simulink model "AC_Voltage_Control_3phase_IM"  (R2025a)
settings: Solver=ode23t  StartTime=0.0  StopTime=5  FixedStep=0.00001  MaxStep=10e-6  RelTol=1e-3  EnableMultiTasking=on
undefined symbols (not defined in the file): DiscIntNeverNeededParam
libraries: spsDetailedThyristorLib x6, spsVoltageMeasurementLib x6, spsACVoltageSourceLib x3, spsAsynchronousMachineSIUnitsLib x1, powerlib_extras x1, spsSeriesRLCBranchLib x1, spsThreePhaseVIMeasurementLib x1, sps_lib x1
settings Model: Creator=jagan  LastModifiedBy=Shubham Raj Gupta
settings SolverCC: ZeroCrossControl=DisableAll  ZeroCrossAlgorithm=Non-adaptive  AlgebraicLoopSolver=TrustRegion
settings DataIOCC: LimitDataPoints=on  SaveFormat=Array  SignalLoggingSaveFormat=ModelDataLogs  ReturnWorkspaceOutputs=off
settings OptimizationCC: ExpressionDepthLimit=2147483647.0  InitFltsAndDblsToZero=on  LifeSpan=inf
settings DebuggingCC: SaveWithParameterizedLinksMsg=none  UnderspecifiedInitializationDetection=Classic  MergeDetectMultiDrivingBlocksExec=none  SignalResolutionControl=TryResolveAllWithWarning  SolverPrmCheckMsg=warning  MultiTaskDSMMsg=warning  MultiTaskCondExecSysMsg=none  FcnCallInpInsideContextMsg=warning  UnconnectedInputMsg=warning  UnconnectedOutputMsg=warning  UnconnectedLineMsg=warning  StateNameClashWarn=warning  SFUnexpectedBacktrackingDiag=warning  SFNoUnconditionalDefaultTransitionDiag=warning  SFExecutionAtInitializationDiag=none  ArithmeticOperatorsInVariantConditions=warning
settings HardwareCC: ProdBitPerPointer=32.0  ProdBitPerSizeT=32.0  ProdBitPerPtrDiffT=32.0  ProdLargestAtomicFloat=None  ProdIntDivRoundTo=Undefined  ProdEndianess=Unspecified  ProdWordSize=32.0  ProdHWDeviceType=32-bit Generic
settings ModelReferenceCC: PropagateSignalLabelsOutOfModel=off
settings SFSimCC: SimParseCustomCode=off
settings RTWCC: GPUComputeCapability=3.5
settings CodeAppCC: StateflowObjectComments=on
settings GRTTargetCC: TargetFcnLib=ansi_tfl_tmw.mat  TargetLangStandard=C89/C90 (ANSI)  CombineOutputUpdateFcns=off  GRTInterface=on
settings ConfigComp: CovMetricSettings=dw  CovSaveCumulativeToWorkspaceVar=on  CovSaveSingleToWorkspaceVar=on

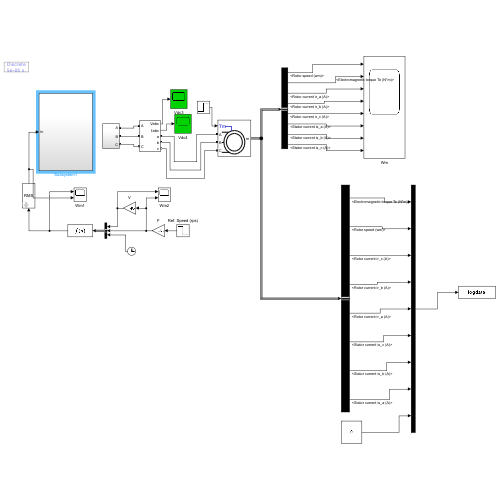
[thumbnail: Simulink's stored preview of the top-level diagram]
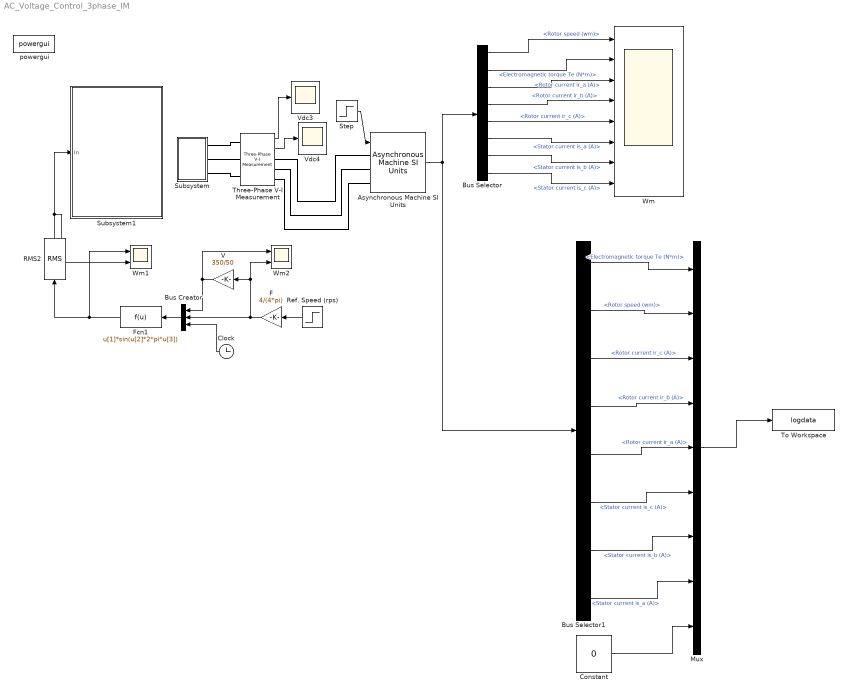
== system AC_Voltage_Control_3phase_IM ==
  Asynchronous Machine SI Units : spsAsynchronousMachineSIUnitsLib/Asynchronous Machine SI Units  RotorType=Squirrel-cage  PresetModel=No  MechanicalLoad=Torque Tm  ShowDetailedParameters=on  ReferenceFrame=Rotor  Units=SI  MeasurementBus=off  NominalParameters=[3730 400 50]  VoltageRatio=1  Stator=[1.115 0.005974]  Rotor=[100 0.005974]  Cage1=[0.4155 0.002066]  Cage2=[0.4168 0.0003495]  Lm=0.2037  Mechanical=[0.02 0.005752 2]  PolePairs=2  InitialConditions="[ 1,0   0,0,0   0,0,0 ]"  SimulateSaturation=off  Saturation=[9.9249,19.6672,38.0377,51.3988,69.2824,105.1337,152.5532,214.2421,303.1917;230, 322, 414, 460, 506, 552, 598, 644, 690]  LoadFlowParameters=0  TsPowergui=0  TsBlock=-1  IterativeModel=Trapezoidal non iterative  IterativeDiscreteModel=Trapezoidal non iterative  Pmec=1.492e+006
  Bus Creator : BusCreator  Inputs=3
  Bus Selector : BusSelector  OutputSignals=Mechanical.Rotor speed (wm),Mechanical.Electromagnetic torque Te (N*m),Rotor measurements.Rotor current ir_a (A),Rotor measurements.Rotor current ir_b (A),Rotor measurements.Rotor current ir_c (A),Stator measurements.Stator current is_a (A),Stator measurements.Stator current is_b (A),Stator measurements.Stator current is_c (A)
  Bus Selector1 : BusSelector  OutputSignals=Mechanical.Electromagnetic torque Te (N*m),Mechanical.Rotor speed (wm),Rotor measurements.Rotor current ir_c (A),Rotor measurements.Rotor current ir_b (A),Rotor measurements.Rotor current ir_a (A),Stator measurements.Stator current is_c (A),Stator measurements.Stator current is_b (A),Stator measurements.Stator current is_a (A)
  Clock : Clock
  Constant : Constant  Value=0
  F : Gain  Gain=4/(4*pi)
  Fcn1 : Fcn  Expr=u[1]*sin(u[2]*2*pi*u[3])
  Mux : Mux  Inputs=9
  RMS2 : powerlib_extras/Measurements/RMS  f1=50
  Ref. Speed (rps) : Step  Time=3  Before=150  After=120  SampleTime=0
  Step : Step  After=3  SampleTime=0
  Subsystem : Subsystem
  Subsystem1 : Subsystem
  Three-Phase V-I Measurement : spsThreePhaseVIMeasurementLib/Three-Phase V-I Measurement  VoltageMeasurement=phase-to-phase  SetLabelV=off  LabelV=Vabc  Vpu=off  VpuLL=off  CurrentMeasurement=yes  SetLabelI=off  LabelI=Iabc  Ipu=off  Pbase=100e6  Vbase=500e3  OutputType=Complex  PhasorSimulation=off  PSBequivalent=0
  To Workspace : ToWorkspace  VariableName=logdata  SampleTime=5e-5
  V : Gain  Gain=350/50
  Vdc3 : Scope
      settings: SampleTime=100e-6  TimeSpan=0.04  ActiveDisplayYMinimum=-700  ActiveDisplayYMaximum=700  DataLoggingVariableName=Ia_3
  Vdc4 : Scope
      settings: SampleTime=100e-6  TimeSpan=1  ActiveDisplayYMinimum=549.65  ActiveDisplayYMaximum=549.82  DataLoggingVariableName=Ia_4
  Wm : Scope  NumInputPorts=8
      settings: ActiveDisplayYMinimum=-300  ActiveDisplayYMaximum=207.4144440126116  DataLoggingVariableName=ScopeData9
  Wm1 : Scope  NumInputPorts=2
      settings: TimeSpan=0.04  ActiveDisplayYMinimum=-350  ActiveDisplayYMaximum=350
  Wm2 : Scope  NumInputPorts=2
      settings: ActiveDisplayYMinimum=332.332  ActiveDisplayYMaximum=367.314  DataLoggingVariableName=ScopeData7
  powergui : sps_lib/powergui  SimulationMode=Discrete  SampleTime=50e-6  frequency=60  Iterations=50  frequencyindice=50  Pbase=100e6  ErrMax=1e-4  UnitsV=kV  UnitsW=MW  buscounter=0  FunctionMessages=off  echomessages=off  EnableUseOfTLC=off  CurrentSourceSwitches=off  DisableSnubberDevices=off  DisableRonSwitches=off  DisableVfSwitches=off  DisplayEquations=off  AutomaticDiscreteSolvers=off  SolverType=Tustin/Backward Euler (TBE)  Interpol=off  ExternalGateDelay=off  methode=off  Ts=0  x0status=blocks  SPID=off  SwTol=0  HookPort=off  NonlinearTolerance=1e-4  nMaxIteration=100  ContinueOnMaxIteration=off  RestoreLinks=warning  ResistiveCurrentMeasurement=off  Frange=[0:2:500]  Ylog=off  Xlog=on  ShowGrid=off  save=off  variable=ZData  structure=0  ZoomFFT=on  StartTime=0.0  cycles=1  DisplayStyle=1  fundamental=60  FreqAxis=off  MaxFrequency=1000  frequencyindicesteady=1  RmsSteady=1  display=off
  wires:
  Bus Creator/1 -> Fcn1/1
  Clock/1 -> Bus Creator/3
  F/1 -> Bus Creator/2, V/1, Wm2/2
  V/1 -> Bus Creator/1, Wm2/1
  Ref. Speed (rps)/1 -> F/1
  Fcn1/1 -> RMS2/1, Wm1/1
  RMS2/1 -> Subsystem1/1(In), Wm1/2
  Step/1 -> Asynchronous Machine SI Units/1
  Asynchronous Machine SI Units/1 -> Bus Selector1/1, Bus Selector/1
  Bus Selector/1 -> Wm/1  "<Rotor speed (wm)>"
  Bus Selector/2 -> Wm/2  "<Electromagnetic torque Te (N*m)>"
  Three-Phase V-I Measurement/1 -> Vdc3/1
  Three-Phase V-I Measurement/2 -> Vdc4/1
  Constant/1 -> Mux/9
  Mux/1 -> To Workspace/1
  Bus Selector1/1 -> Mux/1  "<Electromagnetic torque Te (N*m)>"
  Bus Selector1/2 -> Mux/2  "<Rotor speed (wm)>"
  Bus Selector1/3 -> Mux/3  "<Rotor current ir_c (A)>"
  Bus Selector1/4 -> Mux/4  "<Rotor current ir_b (A)>"
  Bus Selector1/5 -> Mux/5  "<Rotor current ir_a (A)>"
  Bus Selector1/6 -> Mux/6  "<Stator current is_c (A)>"
  Bus Selector1/7 -> Mux/7  "<Stator current is_b (A)>"
  Bus Selector1/8 -> Mux/8  "<Stator current is_a (A)>"
  Bus Selector/3 -> Wm/3  "<Rotor current ir_a (A)>"
  Bus Selector/4 -> Wm/4  "<Rotor current ir_b (A)>"
  Bus Selector/5 -> Wm/5  "<Rotor current ir_c (A)>"
  Bus Selector/6 -> Wm/6  "<Stator current is_a (A)>"
  Bus Selector/7 -> Wm/7  "<Stator current is_b (A)>"
  Bus Selector/8 -> Wm/8  "<Stator current is_c (A)>"
  connections:
  Three-Phase V-I Measurement/LConn1 -- Subsystem/RConn1
  Subsystem/RConn2 -- Three-Phase V-I Measurement/LConn2
  Three-Phase V-I Measurement/LConn3 -- Subsystem/RConn3
  Three-Phase V-I Measurement/RConn1 -- Asynchronous Machine SI Units/LConn1
  Asynchronous Machine SI Units/LConn2 -- Three-Phase V-I Measurement/RConn2
  Three-Phase V-I Measurement/RConn3 -- Asynchronous Machine SI Units/LConn3

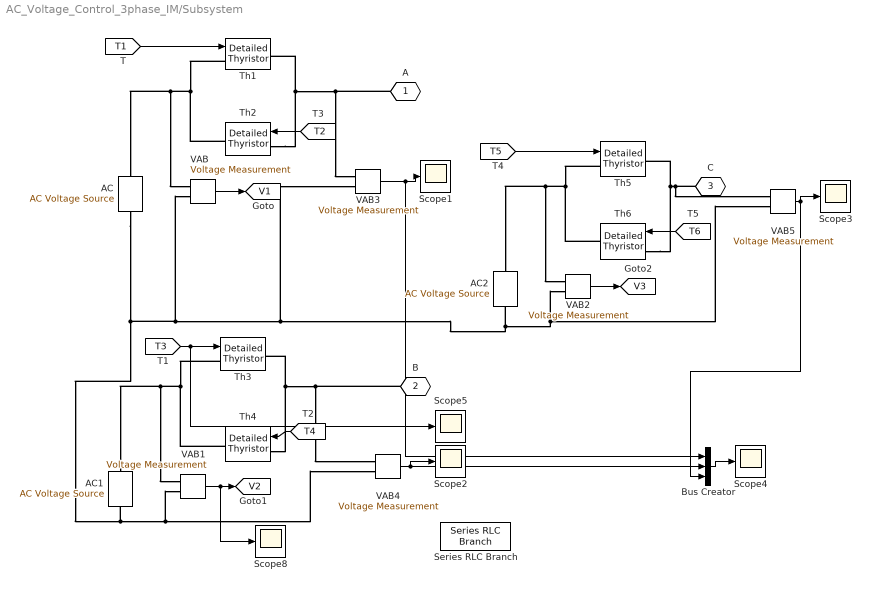
== system AC_Voltage_Control_3phase_IM/Subsystem ==
  AC : spsACVoltageSourceLib/AC Voltage Source  Amplitude=250*1.414  Phase=0  Frequency=50  SampleTime=0  Measurements=None  BusType=swing  Pref=10e3  Qref=0  Qmin=-inf  Qmax=+inf
  AC1 : spsACVoltageSourceLib/AC Voltage Source  Amplitude=250*1.414  Phase=240  Frequency=50  SampleTime=0  Measurements=None  BusType=swing  Pref=10e3  Qref=0  Qmin=-inf  Qmax=+inf
  AC2 : spsACVoltageSourceLib/AC Voltage Source  Amplitude=250*1.414  Phase=120  Frequency=50  SampleTime=0  Measurements=None  BusType=swing  Pref=10e3  Qref=0  Qmin=-inf  Qmax=+inf
  Bus Creator : BusCreator  Inputs=3
  Scope{1..5,8} (6 alike) : Scope
      Scope1 settings: TimeSpan=0.04  ActiveDisplayYMinimum=-300  ActiveDisplayYMaximum=300  DataLoggingVariableName=ScopeData2
      Scope2 settings: TimeSpan=0.04  ActiveDisplayYMinimum=-400  ActiveDisplayYMaximum=400  DataLoggingVariableName=ScopeData3
      Scope3 settings: TimeSpan=0.04  ActiveDisplayYMinimum=-400  ActiveDisplayYMaximum=400  DataLoggingVariableName=ScopeData4
      Scope4 settings: TimeSpan=0.04  ActiveDisplayYMinimum=-400  ActiveDisplayYMaximum=400  DataLoggingVariableName=ScopeData5
      Scope5 settings: TimeSpan=0.04  ActiveDisplayYMinimum=0  ActiveDisplayYMaximum=1  DataLoggingVariableName=ScopeData6
      Scope8 settings: TimeSpan=0.04  ActiveDisplayYMinimum=-400  ActiveDisplayYMaximum=400  DataLoggingVariableName=ScopeData10
  Series RLC Branch : spsSeriesRLCBranchLib/Series RLC Branch  LConnTagsString=__new0  RConnTagsString=__new0  BranchType=RLC  Resistance=1  Inductance=1e-3  SetiL0=off  InitialCurrent=0  Capacitance=1e-6  Setx0=off  InitialVoltage=0  Measurements=None
  Th{1..6} (6 alike) : spsDetailedThyristorLib/Detailed Thyristor  Ron=0.001  Lon=0  Vf=0.8  IL=0.1  Tq=100e-6  IC=0  Rs=500  Cs=250e-9  Measurements=off
      settings: LibrarySourceBlock=sps_lib/Power Electronics/Detailed Thyristor
  VAB{,1..5} (6 alike) : spsVoltageMeasurementLib/Voltage Measurement  PhasorSimulation=off  OutputType=Complex  PSBequivalent=0
  A : PMIOPort  Tag=PMCPort  Side=Right
  B : PMIOPort  Tag=PMCPort  Port=2  Side=Right
  C : PMIOPort  Tag=PMCPort  Port=3  Side=Right
  tag scope: V1=global, V2=global, V3=global
  wires:
  VAB/1 -> [V1]
  [T1] -> Th1/1
  [T2] -> Th2/1
  VAB1/1 -> [V2], Scope8/1
  [T3] -> Scope5/1, Th3/1
  [T4] -> Th4/1
  VAB2/1 -> [V3]
  [T5] -> Th5/1
  [T6] -> Th6/1
  VAB3/1 -> Scope1/1, Bus Creator/1
  VAB4/1 -> Scope2/1, Bus Creator/2
  VAB5/1 -> Scope3/1, Bus Creator/3
  Bus Creator/1 -> Scope4/1
  connections:
  Th1/LConn1 -- AC/RConn1 -- VAB/LConn1 -- Th2/RConn1
  Th4/RConn1 -- VAB1/LConn1 -- AC1/RConn1 -- Th3/LConn1
  Th1/RConn1 -- A/RConn1 -- VAB3/LConn1 -- Th2/LConn1
  Th4/LConn1 -- VAB4/LConn1 -- B/RConn1 -- Th3/RConn1
  Th5/LConn1 -- AC2/RConn1 -- VAB2/LConn1 -- Th6/RConn1
  Th5/RConn1 -- C/RConn1 -- VAB5/LConn1 -- Th6/LConn1
  VAB1/LConn2 -- VAB4/LConn2 -- AC1/LConn1 -- AC/LConn1 -- VAB/LConn2 -- VAB3/LConn2 -- AC2/LConn1 -- VAB2/LConn2 -- VAB5/LConn2

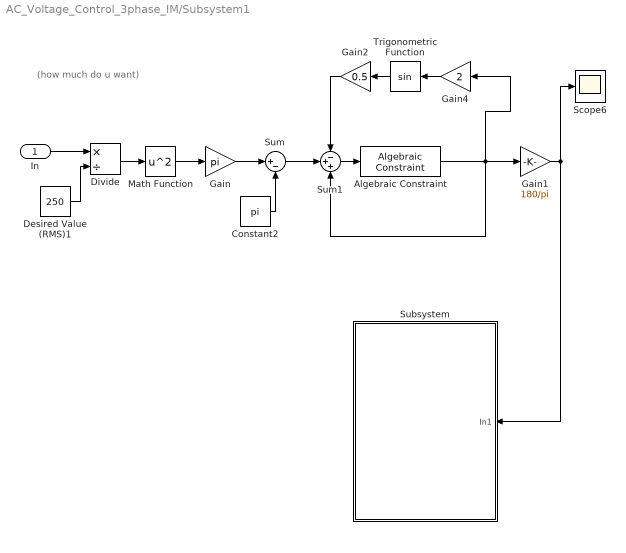
== system AC_Voltage_Control_3phase_IM/Subsystem1 ==
  note: (how much do u want)
  In : Inport
  Algebraic Constraint : AlgebraicConstraint  InitialGuess=pi
  Constant2 : Constant  Value=pi
  Desired Value (RMS)1 : Constant  Value=250
  Divide : Product  Inputs=*/
  Gain : Gain  Gain=pi
  Gain1 : Gain  Gain=180/pi
  Gain2 : Gain  Gain=0.5
  Gain4 : Gain  Gain=2
  Math Function : Math  Operator=square  SignedPower=on
  Scope6 : Scope
      settings: TimeSpan=0.04  ActiveDisplayYMinimum=26.65  ActiveDisplayYMaximum=27.15
  Subsystem : Subsystem
  Sum : Sum  Inputs=|+-
  Sum1 : Sum  Inputs=-++
  Trigonometric Function : Trigonometry  SampleTime=0.0001
  wires:
  In/1 -> Divide/1
  Divide/1 -> Math Function/1
  Math Function/1 -> Gain/1
  Gain/1 -> Sum/1
  Constant2/1 -> Sum/2
  Sum1/1 -> Algebraic Constraint/1
  Algebraic Constraint/1 -> Sum1/3, Gain1/1, Gain4/1
  Gain4/1 -> Trigonometric Function/1
  Trigonometric Function/1 -> Gain2/1
  Gain2/1 -> Sum1/1
  Sum/1 -> Sum1/2
  Gain1/1 -> Scope6/1, Subsystem/1(In1)
  Desired Value (RMS)1/1 -> Divide/2

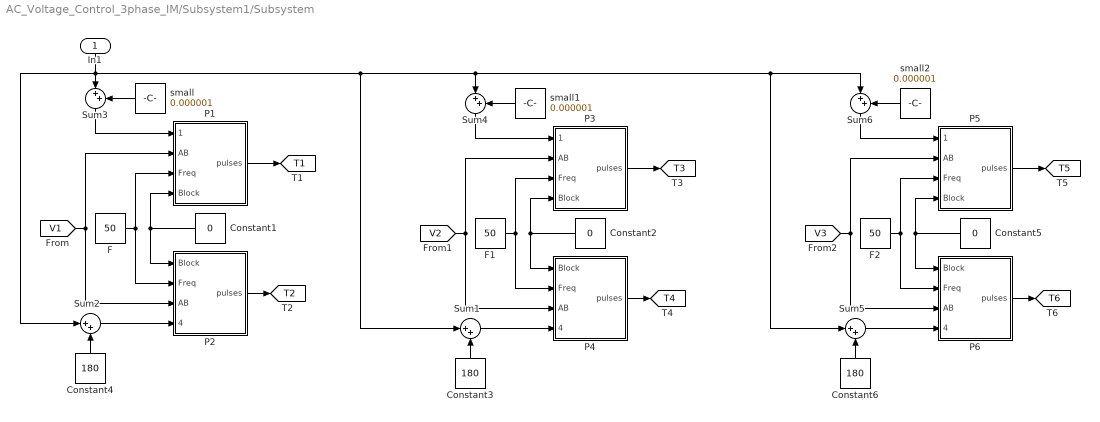
== system AC_Voltage_Control_3phase_IM/Subsystem1/Subsystem ==
  In1 : Inport
  Constant1 : Constant  Value=0
  Constant2 : Constant  Value=0
  Constant3 : Constant  Value=180
  Constant4 : Constant  Value=180
  Constant5 : Constant  Value=0
  Constant6 : Constant  Value=180
  F : Constant  Value=50
  F1 : Constant  Value=50
  F2 : Constant  Value=50
  P1 : Subsystem  AncestorBlock=|  DialogController=POWERSYS.PowerSysDialog  mask(Discrete Synchronized 6-pulse generator){pwidth=10, Double_Pulse=on, Ts=0.0001}
      | powerlib_extras/Discrete 
      | Control Blocks/Discrete Synchronized
      | 6-Pulse Generator
      mask prompts: pwidth "Pulse width (degrees) :"; Double_Pulse "Double pulsing"; Ts "Time step (s) :"
      mask help:
      | Use this block to fire the 6 thyristors of a 6-pulse converter.
      |
      | The output is a vector of 6 pulses (0-1) individually synchronized on the 6 commutation voltages. Pulses are generated alpha degrees after the increasing zero-crossings of the commutation voltages.
      |
      | Input 1 is  the alpha firing signal (degrees).
      | Inputs 2, 3 and 4 are the synchronization voltages AB BC CA which should be in phase with the 3 phase-phase voltages at the converter terminals.
      | Input 5: Frequency of the synchronization voltages (use a constant or the Freq PLL output)
      | Input 6 allows  blocking of the pulses when the applied signal is non zero.
      |
      | When the 'Douple pulsing' option is checked, two pulses are sent to each thyristor: a 1st pulse when the aplha angle is reached, then a 2nd pulse 60 degrees later, when the next thyristor is fired.
      mask init:
      | power_initmask();
      mask Help: This block is part of a subset of blocks in the Extras library that does not have documentation associated with it, other than the block mask description.
      mask Display: plot(0,0,100,100,[80 62 62 47 47 30],[40 40 60 60 40 40]-5)
  P2 : Subsystem  AncestorBlock=|  DialogController=POWERSYS.PowerSysDialog  mask(Discrete Synchronized 6-pulse generator){pwidth=10, Double_Pulse=on, Ts=0.0001}
      | powerlib_extras/Discrete 
      | Control Blocks/Discrete Synchronized
      | 6-Pulse Generator
      mask prompts: pwidth "Pulse width (degrees) :"; Double_Pulse "Double pulsing"; Ts "Time step (s) :"
      mask help:
      | Use this block to fire the 6 thyristors of a 6-pulse converter.
      |
      | The output is a vector of 6 pulses (0-1) individually synchronized on the 6 commutation voltages. Pulses are generated alpha degrees after the increasing zero-crossings of the commutation voltages.
      |
      | Input 1 is  the alpha firing signal (degrees).
      | Inputs 2, 3 and 4 are the synchronization voltages AB BC CA which should be in phase with the 3 phase-phase voltages at the converter terminals.
      | Input 5: Frequency of the synchronization voltages (use a constant or the Freq PLL output)
      | Input 6 allows  blocking of the pulses when the applied signal is non zero.
      |
      | When the 'Douple pulsing' option is checked, two pulses are sent to each thyristor: a 1st pulse when the aplha angle is reached, then a 2nd pulse 60 degrees later, when the next thyristor is fired.
      mask init:
      | power_initmask();
      mask Help: This block is part of a subset of blocks in the Extras library that does not have documentation associated with it, other than the block mask description.
      mask Display: plot(0,0,100,100,[80 62 62 47 47 30],[40 40 60 60 40 40]-5)
  P3 : Subsystem  AncestorBlock=|  DialogController=POWERSYS.PowerSysDialog  mask(Discrete Synchronized 6-pulse generator){pwidth=180, Double_Pulse=on, Ts=0.0001}
      | powerlib_extras/Discrete 
      | Control Blocks/Discrete Synchronized
      | 6-Pulse Generator
      mask prompts: pwidth "Pulse width (degrees) :"; Double_Pulse "Double pulsing"; Ts "Time step (s) :"
      mask help:
      | Use this block to fire the 6 thyristors of a 6-pulse converter.
      |
      | The output is a vector of 6 pulses (0-1) individually synchronized on the 6 commutation voltages. Pulses are generated alpha degrees after the increasing zero-crossings of the commutation voltages.
      |
      | Input 1 is  the alpha firing signal (degrees).
      | Inputs 2, 3 and 4 are the synchronization voltages AB BC CA which should be in phase with the 3 phase-phase voltages at the converter terminals.
      | Input 5: Frequency of the synchronization voltages (use a constant or the Freq PLL output)
      | Input 6 allows  blocking of the pulses when the applied signal is non zero.
      |
      | When the 'Douple pulsing' option is checked, two pulses are sent to each thyristor: a 1st pulse when the aplha angle is reached, then a 2nd pulse 60 degrees later, when the next thyristor is fired.
      mask init:
      | power_initmask();
      mask Help: This block is part of a subset of blocks in the Extras library that does not have documentation associated with it, other than the block mask description.
      mask Display: plot(0,0,100,100,[80 62 62 47 47 30],[40 40 60 60 40 40]-5)
  P4 : Subsystem  AncestorBlock=|  DialogController=POWERSYS.PowerSysDialog  mask(Discrete Synchronized 6-pulse generator){pwidth=180, Double_Pulse=on, Ts=0.0001}
      | powerlib_extras/Discrete 
      | Control Blocks/Discrete Synchronized
      | 6-Pulse Generator
      mask prompts: pwidth "Pulse width (degrees) :"; Double_Pulse "Double pulsing"; Ts "Time step (s) :"
      mask help:
      | Use this block to fire the 6 thyristors of a 6-pulse converter.
      |
      | The output is a vector of 6 pulses (0-1) individually synchronized on the 6 commutation voltages. Pulses are generated alpha degrees after the increasing zero-crossings of the commutation voltages.
      |
      | Input 1 is  the alpha firing signal (degrees).
      | Inputs 2, 3 and 4 are the synchronization voltages AB BC CA which should be in phase with the 3 phase-phase voltages at the converter terminals.
      | Input 5: Frequency of the synchronization voltages (use a constant or the Freq PLL output)
      | Input 6 allows  blocking of the pulses when the applied signal is non zero.
      |
      | When the 'Douple pulsing' option is checked, two pulses are sent to each thyristor: a 1st pulse when the aplha angle is reached, then a 2nd pulse 60 degrees later, when the next thyristor is fired.
      mask init:
      | power_initmask();
      mask Help: This block is part of a subset of blocks in the Extras library that does not have documentation associated with it, other than the block mask description.
      mask Display: plot(0,0,100,100,[80 62 62 47 47 30],[40 40 60 60 40 40]-5)
  P5 : Subsystem  AncestorBlock=|  DialogController=POWERSYS.PowerSysDialog  mask(Discrete Synchronized 6-pulse generator){pwidth=180, Double_Pulse=on, Ts=0.0001}
      | powerlib_extras/Discrete 
      | Control Blocks/Discrete Synchronized
      | 6-Pulse Generator
      mask prompts: pwidth "Pulse width (degrees) :"; Double_Pulse "Double pulsing"; Ts "Time step (s) :"
      mask help:
      | Use this block to fire the 6 thyristors of a 6-pulse converter.
      |
      | The output is a vector of 6 pulses (0-1) individually synchronized on the 6 commutation voltages. Pulses are generated alpha degrees after the increasing zero-crossings of the commutation voltages.
      |
      | Input 1 is  the alpha firing signal (degrees).
      | Inputs 2, 3 and 4 are the synchronization voltages AB BC CA which should be in phase with the 3 phase-phase voltages at the converter terminals.
      | Input 5: Frequency of the synchronization voltages (use a constant or the Freq PLL output)
      | Input 6 allows  blocking of the pulses when the applied signal is non zero.
      |
      | When the 'Douple pulsing' option is checked, two pulses are sent to each thyristor: a 1st pulse when the aplha angle is reached, then a 2nd pulse 60 degrees later, when the next thyristor is fired.
      mask init:
      | power_initmask();
      mask Help: This block is part of a subset of blocks in the Extras library that does not have documentation associated with it, other than the block mask description.
      mask Display: plot(0,0,100,100,[80 62 62 47 47 30],[40 40 60 60 40 40]-5)
  P6 : Subsystem  AncestorBlock=|  DialogController=POWERSYS.PowerSysDialog  mask(Discrete Synchronized 6-pulse generator){pwidth=180, Double_Pulse=on, Ts=0.0001}
      | powerlib_extras/Discrete 
      | Control Blocks/Discrete Synchronized
      | 6-Pulse Generator
      mask prompts: pwidth "Pulse width (degrees) :"; Double_Pulse "Double pulsing"; Ts "Time step (s) :"
      mask help:
      | Use this block to fire the 6 thyristors of a 6-pulse converter.
      |
      | The output is a vector of 6 pulses (0-1) individually synchronized on the 6 commutation voltages. Pulses are generated alpha degrees after the increasing zero-crossings of the commutation voltages.
      |
      | Input 1 is  the alpha firing signal (degrees).
      | Inputs 2, 3 and 4 are the synchronization voltages AB BC CA which should be in phase with the 3 phase-phase voltages at the converter terminals.
      | Input 5: Frequency of the synchronization voltages (use a constant or the Freq PLL output)
      | Input 6 allows  blocking of the pulses when the applied signal is non zero.
      |
      | When the 'Douple pulsing' option is checked, two pulses are sent to each thyristor: a 1st pulse when the aplha angle is reached, then a 2nd pulse 60 degrees later, when the next thyristor is fired.
      mask init:
      | power_initmask();
      mask Help: This block is part of a subset of blocks in the Extras library that does not have documentation associated with it, other than the block mask description.
      mask Display: plot(0,0,100,100,[80 62 62 47 47 30],[40 40 60 60 40 40]-5)
  Sum{1..6} (6 alike) : Sum  Inputs=|++
  small : Constant  Value=0.000001
  small1 : Constant  Value=0.000001
  small2 : Constant  Value=0.000001
  tag scope: T1=global, T2=global, T3=global, T4=global, T5=global, T6=global
  wires:
  Constant4/1 -> Sum2/2
  small/1 -> Sum3/2
  Sum3/1 -> P1/1(alpha_deg)
  Constant1/1 -> P1/4(Block), P2/1(Block)
  F/1 -> P1/3(Freq), P2/2(Freq)
  Sum2/1 -> P2/4(alpha_deg)
  [V1] -> P1/2(AB), P2/3(AB)
  P1/1(pulses) -> [T1]
  P2/1(pulses) -> [T2]
  In1/1 -> Sum3/1, Sum1/1, Sum4/1, Sum6/1, Sum5/1, Sum2/1
  Constant3/1 -> Sum1/2
  small1/1 -> Sum4/2
  Sum4/1 -> P3/1(alpha_deg)
  Constant2/1 -> P4/1(Block), P3/4(Block)
  F1/1 -> P4/2(Freq), P3/3(Freq)
  Sum1/1 -> P4/4(alpha_deg)
  [V2] -> P4/3(AB), P3/2(AB)
  P3/1(pulses) -> [T3]
  P4/1(pulses) -> [T4]
  Constant6/1 -> Sum5/2
  small2/1 -> Sum6/2
  Sum6/1 -> P5/1(alpha_deg)
  Constant5/1 -> P5/4(Block), P6/1(Block)
  F2/1 -> P5/3(Freq), P6/2(Freq)
  Sum5/1 -> P6/4(alpha_deg)
  [V3] -> P5/2(AB), P6/3(AB)
  P5/1(pulses) -> [T5]
  P6/1(pulses) -> [T6]

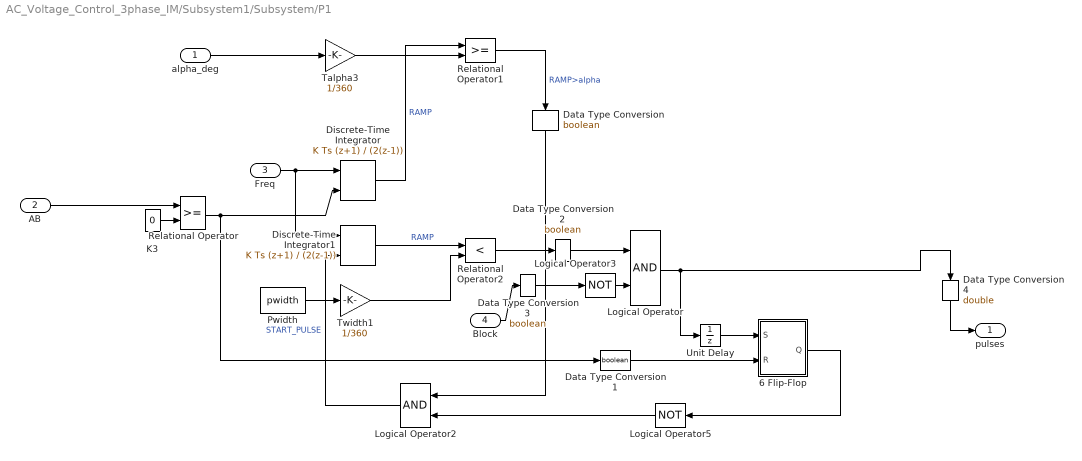
== system AC_Voltage_Control_3phase_IM/Subsystem1/Subsystem/P1 ==
  alpha_deg : Inport
  AB : Inport  Port=2
  Freq : Inport  Port=3
  Block : Inport  Port=4
  6 Flip-Flop : Subsystem
  Data Type Conversion{,1..3} (4 alike) : DataTypeConversion  OutDataTypeStr=boolean
  Data Type Conversion4 : DataTypeConversion  OutDataTypeStr=double
  Discrete-Time Integrator : DiscreteIntegrator  IntegratorMethod=Integration: Trapezoidal  ExternalReset=rising  SampleTime=Ts  ICPrevOutput=DiscIntNeverNeededParam  ICPrevScaledInput=DiscIntNeverNeededParam
  Discrete-Time Integrator1 : DiscreteIntegrator  IntegratorMethod=Integration: Trapezoidal  ExternalReset=rising  SampleTime=Ts  ICPrevOutput=DiscIntNeverNeededParam  ICPrevScaledInput=DiscIntNeverNeededParam
  K3 : Constant  Value=0
  Logical Operator : Logic
  Logical Operator2 : Logic
  Logical Operator3 : Logic  Operator=NOT  Inputs=1
  Logical Operator5 : Logic  Operator=NOT  Inputs=1
  Pwidth : Constant  Value=pwidth
  Relational Operator : RelationalOperator
  Relational Operator1 : RelationalOperator
  Relational Operator2 : RelationalOperator  Operator=<
  Talpha3 : Gain  Gain=1/360  SaturateOnIntegerOverflow=on  OutDataTypeStr=Inherit: Same as input  ParamDataTypeStr=Inherit: Same as input
  Twidth1 : Gain  Gain=1/360  SaturateOnIntegerOverflow=on  OutDataTypeStr=Inherit: Same as input  ParamDataTypeStr=Inherit: Same as input
  Unit Delay : UnitDelay  SampleTime=Ts
  pulses : Outport  InitialOutput=0
  wires:
  Data Type Conversion4/1 -> pulses/1
  Data Type Conversion3/1 -> Logical Operator3/1
  Block/1 -> Data Type Conversion3/1
  Data Type Conversion2/1 -> Logical Operator/1
  Relational Operator2/1 -> Data Type Conversion2/1
  Data Type Conversion1/1 -> 6 Flip-Flop/2(R)
  Data Type Conversion/1 -> Logical Operator2/1
  Relational Operator1/1 -> Data Type Conversion/1  "RAMP>alpha"
  Logical Operator2/1 -> Discrete-Time Integrator1/2  "START_PULSE"
  Logical Operator3/1 -> Logical Operator/2
  Unit Delay/1 -> 6 Flip-Flop/1(S)
  Logical Operator/1 -> Unit Delay/1, Data Type Conversion4/1
  Pwidth/1 -> Twidth1/1
  Twidth1/1 -> Relational Operator2/2
  Discrete-Time Integrator1/1 -> Relational Operator2/1  "RAMP"
  Discrete-Time Integrator/1 -> Relational Operator1/1  "RAMP"
  K3/1 -> Relational Operator/2
  Relational Operator/1 -> Data Type Conversion1/1, Discrete-Time Integrator/2
  Logical Operator5/1 -> Logical Operator2/2
  Talpha3/1 -> Relational Operator1/2
  Freq/1 -> Discrete-Time Integrator/1, Discrete-Time Integrator1/1
  6 Flip-Flop/1(Q) -> Logical Operator5/1
  alpha_deg/1 -> Talpha3/1
  AB/1 -> Relational Operator/1

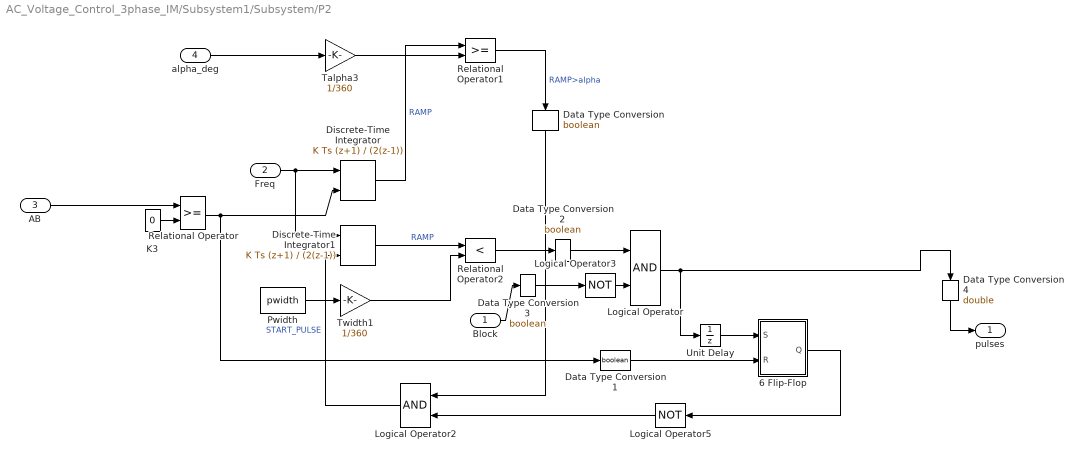
== system AC_Voltage_Control_3phase_IM/Subsystem1/Subsystem/P2 ==
  Block : Inport
  Freq : Inport  Port=2
  AB : Inport  Port=3
  alpha_deg : Inport  Port=4
  6 Flip-Flop : Subsystem
  Data Type Conversion{,1..3} (4 alike) : DataTypeConversion  OutDataTypeStr=boolean
  Data Type Conversion4 : DataTypeConversion  OutDataTypeStr=double
  Discrete-Time Integrator : DiscreteIntegrator  IntegratorMethod=Integration: Trapezoidal  ExternalReset=rising  SampleTime=Ts  ICPrevOutput=DiscIntNeverNeededParam  ICPrevScaledInput=DiscIntNeverNeededParam
  Discrete-Time Integrator1 : DiscreteIntegrator  IntegratorMethod=Integration: Trapezoidal  ExternalReset=rising  SampleTime=Ts  ICPrevOutput=DiscIntNeverNeededParam  ICPrevScaledInput=DiscIntNeverNeededParam
  K3 : Constant  Value=0
  Logical Operator : Logic
  Logical Operator2 : Logic
  Logical Operator3 : Logic  Operator=NOT  Inputs=1
  Logical Operator5 : Logic  Operator=NOT  Inputs=1
  Pwidth : Constant  Value=pwidth
  Relational Operator : RelationalOperator
  Relational Operator1 : RelationalOperator
  Relational Operator2 : RelationalOperator  Operator=<
  Talpha3 : Gain  Gain=1/360  SaturateOnIntegerOverflow=on  OutDataTypeStr=Inherit: Same as input  ParamDataTypeStr=Inherit: Same as input
  Twidth1 : Gain  Gain=1/360  SaturateOnIntegerOverflow=on  OutDataTypeStr=Inherit: Same as input  ParamDataTypeStr=Inherit: Same as input
  Unit Delay : UnitDelay  SampleTime=Ts
  pulses : Outport  InitialOutput=0
  wires:
  AB/1 -> Relational Operator/1
  alpha_deg/1 -> Talpha3/1
  6 Flip-Flop/1(Q) -> Logical Operator5/1
  Freq/1 -> Discrete-Time Integrator1/1, Discrete-Time Integrator/1
  Talpha3/1 -> Relational Operator1/2
  Logical Operator5/1 -> Logical Operator2/2
  Relational Operator/1 -> Discrete-Time Integrator/2, Data Type Conversion1/1
  K3/1 -> Relational Operator/2
  Discrete-Time Integrator/1 -> Relational Operator1/1  "RAMP"
  Discrete-Time Integrator1/1 -> Relational Operator2/1  "RAMP"
  Twidth1/1 -> Relational Operator2/2
  Pwidth/1 -> Twidth1/1
  Logical Operator/1 -> Data Type Conversion4/1, Unit Delay/1
  Unit Delay/1 -> 6 Flip-Flop/1(S)
  Logical Operator3/1 -> Logical Operator/2
  Logical Operator2/1 -> Discrete-Time Integrator1/2  "START_PULSE"
  Relational Operator1/1 -> Data Type Conversion/1  "RAMP>alpha"
  Data Type Conversion/1 -> Logical Operator2/1
  Data Type Conversion1/1 -> 6 Flip-Flop/2(R)
  Relational Operator2/1 -> Data Type Conversion2/1
  Data Type Conversion2/1 -> Logical Operator/1
  Block/1 -> Data Type Conversion3/1
  Data Type Conversion3/1 -> Logical Operator3/1
  Data Type Conversion4/1 -> pulses/1

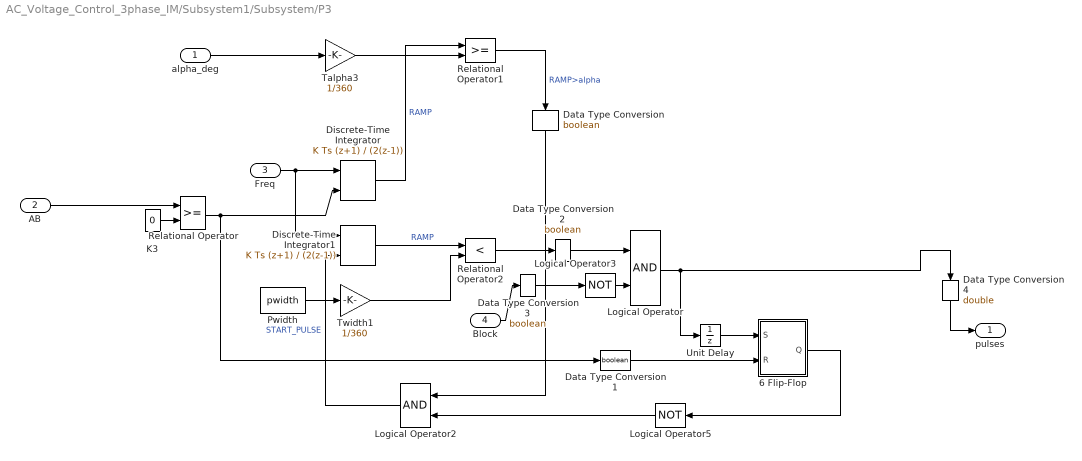
== system AC_Voltage_Control_3phase_IM/Subsystem1/Subsystem/P3 ==
  alpha_deg : Inport
  AB : Inport  Port=2
  Freq : Inport  Port=3
  Block : Inport  Port=4
  6 Flip-Flop : Subsystem
  Data Type Conversion{,1..3} (4 alike) : DataTypeConversion  OutDataTypeStr=boolean
  Data Type Conversion4 : DataTypeConversion  OutDataTypeStr=double
  Discrete-Time Integrator : DiscreteIntegrator  IntegratorMethod=Integration: Trapezoidal  ExternalReset=rising  SampleTime=Ts  ICPrevOutput=DiscIntNeverNeededParam  ICPrevScaledInput=DiscIntNeverNeededParam
  Discrete-Time Integrator1 : DiscreteIntegrator  IntegratorMethod=Integration: Trapezoidal  ExternalReset=rising  SampleTime=Ts  ICPrevOutput=DiscIntNeverNeededParam  ICPrevScaledInput=DiscIntNeverNeededParam
  K3 : Constant  Value=0
  Logical Operator : Logic
  Logical Operator2 : Logic
  Logical Operator3 : Logic  Operator=NOT  Inputs=1
  Logical Operator5 : Logic  Operator=NOT  Inputs=1
  Pwidth : Constant  Value=pwidth
  Relational Operator : RelationalOperator
  Relational Operator1 : RelationalOperator
  Relational Operator2 : RelationalOperator  Operator=<
  Talpha3 : Gain  Gain=1/360  SaturateOnIntegerOverflow=on  OutDataTypeStr=Inherit: Same as input  ParamDataTypeStr=Inherit: Same as input
  Twidth1 : Gain  Gain=1/360  SaturateOnIntegerOverflow=on  OutDataTypeStr=Inherit: Same as input  ParamDataTypeStr=Inherit: Same as input
  Unit Delay : UnitDelay  SampleTime=Ts
  pulses : Outport  InitialOutput=0
  wires:
  AB/1 -> Relational Operator/1
  alpha_deg/1 -> Talpha3/1
  6 Flip-Flop/1(Q) -> Logical Operator5/1
  Freq/1 -> Discrete-Time Integrator1/1, Discrete-Time Integrator/1
  Talpha3/1 -> Relational Operator1/2
  Logical Operator5/1 -> Logical Operator2/2
  Relational Operator/1 -> Discrete-Time Integrator/2, Data Type Conversion1/1
  K3/1 -> Relational Operator/2
  Discrete-Time Integrator/1 -> Relational Operator1/1  "RAMP"
  Discrete-Time Integrator1/1 -> Relational Operator2/1  "RAMP"
  Twidth1/1 -> Relational Operator2/2
  Pwidth/1 -> Twidth1/1
  Logical Operator/1 -> Data Type Conversion4/1, Unit Delay/1
  Unit Delay/1 -> 6 Flip-Flop/1(S)
  Logical Operator3/1 -> Logical Operator/2
  Logical Operator2/1 -> Discrete-Time Integrator1/2  "START_PULSE"
  Relational Operator1/1 -> Data Type Conversion/1  "RAMP>alpha"
  Data Type Conversion/1 -> Logical Operator2/1
  Data Type Conversion1/1 -> 6 Flip-Flop/2(R)
  Relational Operator2/1 -> Data Type Conversion2/1
  Data Type Conversion2/1 -> Logical Operator/1
  Block/1 -> Data Type Conversion3/1
  Data Type Conversion3/1 -> Logical Operator3/1
  Data Type Conversion4/1 -> pulses/1

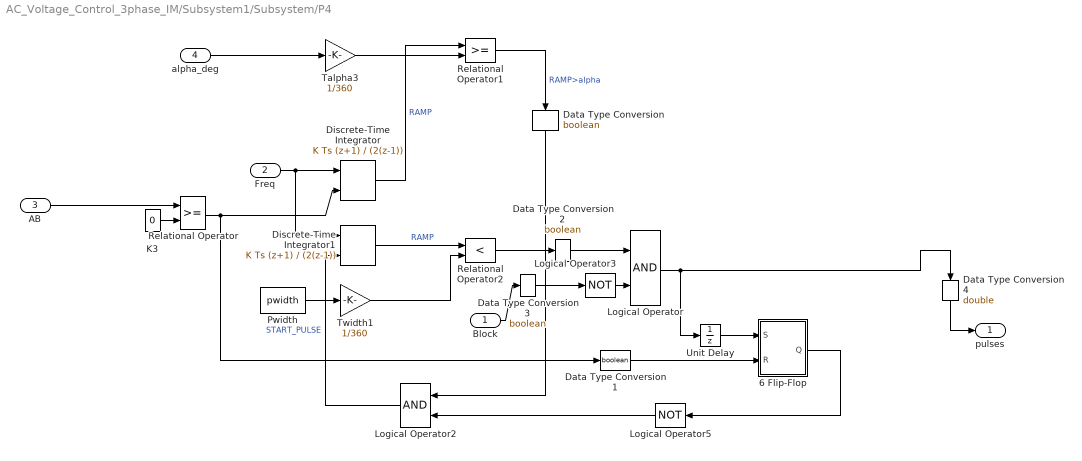
== system AC_Voltage_Control_3phase_IM/Subsystem1/Subsystem/P4 ==
  Block : Inport
  Freq : Inport  Port=2
  AB : Inport  Port=3
  alpha_deg : Inport  Port=4
  6 Flip-Flop : Subsystem
  Data Type Conversion{,1..3} (4 alike) : DataTypeConversion  OutDataTypeStr=boolean
  Data Type Conversion4 : DataTypeConversion  OutDataTypeStr=double
  Discrete-Time Integrator : DiscreteIntegrator  IntegratorMethod=Integration: Trapezoidal  ExternalReset=rising  SampleTime=Ts  ICPrevOutput=DiscIntNeverNeededParam  ICPrevScaledInput=DiscIntNeverNeededParam
  Discrete-Time Integrator1 : DiscreteIntegrator  IntegratorMethod=Integration: Trapezoidal  ExternalReset=rising  SampleTime=Ts  ICPrevOutput=DiscIntNeverNeededParam  ICPrevScaledInput=DiscIntNeverNeededParam
  K3 : Constant  Value=0
  Logical Operator : Logic
  Logical Operator2 : Logic
  Logical Operator3 : Logic  Operator=NOT  Inputs=1
  Logical Operator5 : Logic  Operator=NOT  Inputs=1
  Pwidth : Constant  Value=pwidth
  Relational Operator : RelationalOperator
  Relational Operator1 : RelationalOperator
  Relational Operator2 : RelationalOperator  Operator=<
  Talpha3 : Gain  Gain=1/360  SaturateOnIntegerOverflow=on  OutDataTypeStr=Inherit: Same as input  ParamDataTypeStr=Inherit: Same as input
  Twidth1 : Gain  Gain=1/360  SaturateOnIntegerOverflow=on  OutDataTypeStr=Inherit: Same as input  ParamDataTypeStr=Inherit: Same as input
  Unit Delay : UnitDelay  SampleTime=Ts
  pulses : Outport  InitialOutput=0
  wires:
  Data Type Conversion4/1 -> pulses/1
  Data Type Conversion3/1 -> Logical Operator3/1
  Block/1 -> Data Type Conversion3/1
  Data Type Conversion2/1 -> Logical Operator/1
  Relational Operator2/1 -> Data Type Conversion2/1
  Data Type Conversion1/1 -> 6 Flip-Flop/2(R)
  Data Type Conversion/1 -> Logical Operator2/1
  Relational Operator1/1 -> Data Type Conversion/1  "RAMP>alpha"
  Logical Operator2/1 -> Discrete-Time Integrator1/2  "START_PULSE"
  Logical Operator3/1 -> Logical Operator/2
  Unit Delay/1 -> 6 Flip-Flop/1(S)
  Logical Operator/1 -> Unit Delay/1, Data Type Conversion4/1
  Pwidth/1 -> Twidth1/1
  Twidth1/1 -> Relational Operator2/2
  Discrete-Time Integrator1/1 -> Relational Operator2/1  "RAMP"
  Discrete-Time Integrator/1 -> Relational Operator1/1  "RAMP"
  K3/1 -> Relational Operator/2
  Relational Operator/1 -> Data Type Conversion1/1, Discrete-Time Integrator/2
  Logical Operator5/1 -> Logical Operator2/2
  Talpha3/1 -> Relational Operator1/2
  Freq/1 -> Discrete-Time Integrator/1, Discrete-Time Integrator1/1
  6 Flip-Flop/1(Q) -> Logical Operator5/1
  alpha_deg/1 -> Talpha3/1
  AB/1 -> Relational Operator/1

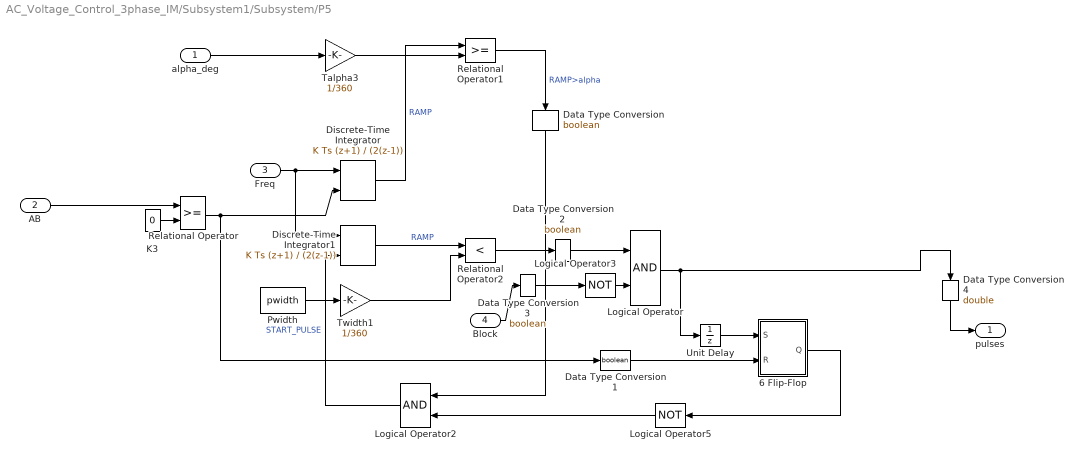
== system AC_Voltage_Control_3phase_IM/Subsystem1/Subsystem/P5 ==
  alpha_deg : Inport
  AB : Inport  Port=2
  Freq : Inport  Port=3
  Block : Inport  Port=4
  6 Flip-Flop : Subsystem
  Data Type Conversion{,1..3} (4 alike) : DataTypeConversion  OutDataTypeStr=boolean
  Data Type Conversion4 : DataTypeConversion  OutDataTypeStr=double
  Discrete-Time Integrator : DiscreteIntegrator  IntegratorMethod=Integration: Trapezoidal  ExternalReset=rising  SampleTime=Ts  ICPrevOutput=DiscIntNeverNeededParam  ICPrevScaledInput=DiscIntNeverNeededParam
  Discrete-Time Integrator1 : DiscreteIntegrator  IntegratorMethod=Integration: Trapezoidal  ExternalReset=rising  SampleTime=Ts  ICPrevOutput=DiscIntNeverNeededParam  ICPrevScaledInput=DiscIntNeverNeededParam
  K3 : Constant  Value=0
  Logical Operator : Logic
  Logical Operator2 : Logic
  Logical Operator3 : Logic  Operator=NOT  Inputs=1
  Logical Operator5 : Logic  Operator=NOT  Inputs=1
  Pwidth : Constant  Value=pwidth
  Relational Operator : RelationalOperator
  Relational Operator1 : RelationalOperator
  Relational Operator2 : RelationalOperator  Operator=<
  Talpha3 : Gain  Gain=1/360  SaturateOnIntegerOverflow=on  OutDataTypeStr=Inherit: Same as input  ParamDataTypeStr=Inherit: Same as input
  Twidth1 : Gain  Gain=1/360  SaturateOnIntegerOverflow=on  OutDataTypeStr=Inherit: Same as input  ParamDataTypeStr=Inherit: Same as input
  Unit Delay : UnitDelay  SampleTime=Ts
  pulses : Outport  InitialOutput=0
  wires:
  Data Type Conversion4/1 -> pulses/1
  Data Type Conversion3/1 -> Logical Operator3/1
  Block/1 -> Data Type Conversion3/1
  Data Type Conversion2/1 -> Logical Operator/1
  Relational Operator2/1 -> Data Type Conversion2/1
  Data Type Conversion1/1 -> 6 Flip-Flop/2(R)
  Data Type Conversion/1 -> Logical Operator2/1
  Relational Operator1/1 -> Data Type Conversion/1  "RAMP>alpha"
  Logical Operator2/1 -> Discrete-Time Integrator1/2  "START_PULSE"
  Logical Operator3/1 -> Logical Operator/2
  Unit Delay/1 -> 6 Flip-Flop/1(S)
  Logical Operator/1 -> Unit Delay/1, Data Type Conversion4/1
  Pwidth/1 -> Twidth1/1
  Twidth1/1 -> Relational Operator2/2
  Discrete-Time Integrator1/1 -> Relational Operator2/1  "RAMP"
  Discrete-Time Integrator/1 -> Relational Operator1/1  "RAMP"
  K3/1 -> Relational Operator/2
  Relational Operator/1 -> Data Type Conversion1/1, Discrete-Time Integrator/2
  Logical Operator5/1 -> Logical Operator2/2
  Talpha3/1 -> Relational Operator1/2
  Freq/1 -> Discrete-Time Integrator/1, Discrete-Time Integrator1/1
  6 Flip-Flop/1(Q) -> Logical Operator5/1
  alpha_deg/1 -> Talpha3/1
  AB/1 -> Relational Operator/1

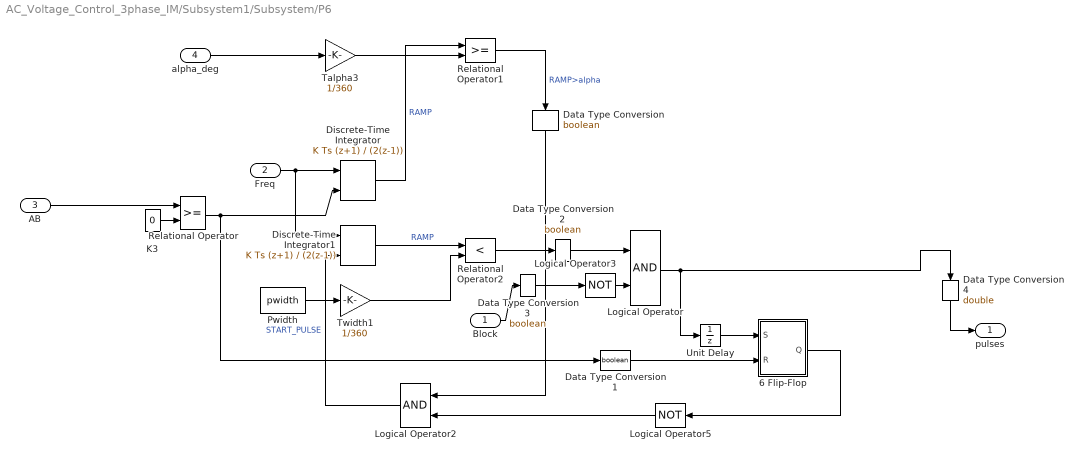
== system AC_Voltage_Control_3phase_IM/Subsystem1/Subsystem/P6 ==
  Block : Inport
  Freq : Inport  Port=2
  AB : Inport  Port=3
  alpha_deg : Inport  Port=4
  6 Flip-Flop : Subsystem
  Data Type Conversion{,1..3} (4 alike) : DataTypeConversion  OutDataTypeStr=boolean
  Data Type Conversion4 : DataTypeConversion  OutDataTypeStr=double
  Discrete-Time Integrator : DiscreteIntegrator  IntegratorMethod=Integration: Trapezoidal  ExternalReset=rising  SampleTime=Ts  ICPrevOutput=DiscIntNeverNeededParam  ICPrevScaledInput=DiscIntNeverNeededParam
  Discrete-Time Integrator1 : DiscreteIntegrator  IntegratorMethod=Integration: Trapezoidal  ExternalReset=rising  SampleTime=Ts  ICPrevOutput=DiscIntNeverNeededParam  ICPrevScaledInput=DiscIntNeverNeededParam
  K3 : Constant  Value=0
  Logical Operator : Logic
  Logical Operator2 : Logic
  Logical Operator3 : Logic  Operator=NOT  Inputs=1
  Logical Operator5 : Logic  Operator=NOT  Inputs=1
  Pwidth : Constant  Value=pwidth
  Relational Operator : RelationalOperator
  Relational Operator1 : RelationalOperator
  Relational Operator2 : RelationalOperator  Operator=<
  Talpha3 : Gain  Gain=1/360  SaturateOnIntegerOverflow=on  OutDataTypeStr=Inherit: Same as input  ParamDataTypeStr=Inherit: Same as input
  Twidth1 : Gain  Gain=1/360  SaturateOnIntegerOverflow=on  OutDataTypeStr=Inherit: Same as input  ParamDataTypeStr=Inherit: Same as input
  Unit Delay : UnitDelay  SampleTime=Ts
  pulses : Outport  InitialOutput=0
  wires:
  AB/1 -> Relational Operator/1
  alpha_deg/1 -> Talpha3/1
  6 Flip-Flop/1(Q) -> Logical Operator5/1
  Freq/1 -> Discrete-Time Integrator1/1, Discrete-Time Integrator/1
  Talpha3/1 -> Relational Operator1/2
  Logical Operator5/1 -> Logical Operator2/2
  Relational Operator/1 -> Discrete-Time Integrator/2, Data Type Conversion1/1
  K3/1 -> Relational Operator/2
  Discrete-Time Integrator/1 -> Relational Operator1/1  "RAMP"
  Discrete-Time Integrator1/1 -> Relational Operator2/1  "RAMP"
  Twidth1/1 -> Relational Operator2/2
  Pwidth/1 -> Twidth1/1
  Logical Operator/1 -> Data Type Conversion4/1, Unit Delay/1
  Unit Delay/1 -> 6 Flip-Flop/1(S)
  Logical Operator3/1 -> Logical Operator/2
  Logical Operator2/1 -> Discrete-Time Integrator1/2  "START_PULSE"
  Relational Operator1/1 -> Data Type Conversion/1  "RAMP>alpha"
  Data Type Conversion/1 -> Logical Operator2/1
  Data Type Conversion1/1 -> 6 Flip-Flop/2(R)
  Relational Operator2/1 -> Data Type Conversion2/1
  Data Type Conversion2/1 -> Logical Operator/1
  Block/1 -> Data Type Conversion3/1
  Data Type Conversion3/1 -> Logical Operator3/1
  Data Type Conversion4/1 -> pulses/1

== system AC_Voltage_Control_3phase_IM/Subsystem1/Subsystem/P1/6 Flip-Flop ==
  S : Inport
  R : Inport  Port=2
  S-R Flip-Flop1 : Subsystem  mask(SRFlipFlop){initial_condition=0, Ts=Ts}
      mask prompts: initial_condition "Initial condition:"; Ts "Sample time:"
      mask help: S-R Flip Flop Block
  Terminator : Terminator
  Q : Outport
  wires:
  S-R Flip-Flop1/1(Q) -> Q/1
  S-R Flip-Flop1/2(!Q) -> Terminator/1
  S/1 -> S-R Flip-Flop1/1(S)
  R/1 -> S-R Flip-Flop1/2(R)

== system AC_Voltage_Control_3phase_IM/Subsystem1/Subsystem/P2/6 Flip-Flop ==
  S : Inport
  R : Inport  Port=2
  S-R Flip-Flop1 : Subsystem  mask(SRFlipFlop){initial_condition=0, Ts=Ts}
      mask prompts: initial_condition "Initial condition:"; Ts "Sample time:"
      mask help: S-R Flip Flop Block
  Terminator : Terminator
  Q : Outport
  wires:
  R/1 -> S-R Flip-Flop1/2(R)
  S/1 -> S-R Flip-Flop1/1(S)
  S-R Flip-Flop1/2(!Q) -> Terminator/1
  S-R Flip-Flop1/1(Q) -> Q/1

== system AC_Voltage_Control_3phase_IM/Subsystem1/Subsystem/P3/6 Flip-Flop ==
  S : Inport
  R : Inport  Port=2
  S-R Flip-Flop1 : Subsystem  mask(SRFlipFlop){initial_condition=0, Ts=Ts}
      mask prompts: initial_condition "Initial condition:"; Ts "Sample time:"
      mask help: S-R Flip Flop Block
  Terminator : Terminator
  Q : Outport
  wires:
  R/1 -> S-R Flip-Flop1/2(R)
  S/1 -> S-R Flip-Flop1/1(S)
  S-R Flip-Flop1/2(!Q) -> Terminator/1
  S-R Flip-Flop1/1(Q) -> Q/1

== system AC_Voltage_Control_3phase_IM/Subsystem1/Subsystem/P4/6 Flip-Flop ==
  S : Inport
  R : Inport  Port=2
  S-R Flip-Flop1 : Subsystem  mask(SRFlipFlop){initial_condition=0, Ts=Ts}
      mask prompts: initial_condition "Initial condition:"; Ts "Sample time:"
      mask help: S-R Flip Flop Block
  Terminator : Terminator
  Q : Outport
  wires:
  S-R Flip-Flop1/1(Q) -> Q/1
  S-R Flip-Flop1/2(!Q) -> Terminator/1
  S/1 -> S-R Flip-Flop1/1(S)
  R/1 -> S-R Flip-Flop1/2(R)

== system AC_Voltage_Control_3phase_IM/Subsystem1/Subsystem/P5/6 Flip-Flop ==
  S : Inport
  R : Inport  Port=2
  S-R Flip-Flop1 : Subsystem  mask(SRFlipFlop){initial_condition=0, Ts=Ts}
      mask prompts: initial_condition "Initial condition:"; Ts "Sample time:"
      mask help: S-R Flip Flop Block
  Terminator : Terminator
  Q : Outport
  wires:
  S-R Flip-Flop1/1(Q) -> Q/1
  S-R Flip-Flop1/2(!Q) -> Terminator/1
  S/1 -> S-R Flip-Flop1/1(S)
  R/1 -> S-R Flip-Flop1/2(R)

== system AC_Voltage_Control_3phase_IM/Subsystem1/Subsystem/P6/6 Flip-Flop ==
  S : Inport
  R : Inport  Port=2
  S-R Flip-Flop1 : Subsystem  mask(SRFlipFlop){initial_condition=0, Ts=Ts}
      mask prompts: initial_condition "Initial condition:"; Ts "Sample time:"
      mask help: S-R Flip Flop Block
  Terminator : Terminator
  Q : Outport
  wires:
  R/1 -> S-R Flip-Flop1/2(R)
  S/1 -> S-R Flip-Flop1/1(S)
  S-R Flip-Flop1/2(!Q) -> Terminator/1
  S-R Flip-Flop1/1(Q) -> Q/1

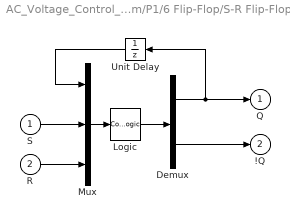
== system AC_Voltage_Control_3phase_IM/Subsystem1/Subsystem/P1/6 Flip-Flop/S-R Flip-Flop1 ==
  S : Inport
  R : Inport  Port=2
  Demux : Demux  Outputs=2
      settings: DisplayOption=none
  Logic : CombinatorialLogic  TruthTable=[0 1;0 1;1 0;0 1;1 0;0 1;1 0;1 0]
  Mux : Mux  Inputs=3
  Unit Delay : UnitDelay  InitialCondition=initial_condition  SampleTime=Ts
  Q : Outport  InitialOutput=0
  !Q : Outport  Port=2  InitialOutput=1
  wires:
  R/1 -> Mux/3
  S/1 -> Mux/2
  Unit Delay/1 -> Mux/1
  Demux/1 -> Unit Delay/1, Q/1
  Demux/2 -> !Q/1
  Logic/1 -> Demux/1
  Mux/1 -> Logic/1

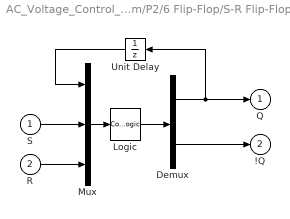
== system AC_Voltage_Control_3phase_IM/Subsystem1/Subsystem/P2/6 Flip-Flop/S-R Flip-Flop1 ==
  S : Inport
  R : Inport  Port=2
  Demux : Demux  Outputs=2
      settings: DisplayOption=none
  Logic : CombinatorialLogic  TruthTable=[0 1;0 1;1 0;0 1;1 0;0 1;1 0;1 0]
  Mux : Mux  Inputs=3
  Unit Delay : UnitDelay  InitialCondition=initial_condition  SampleTime=Ts
  Q : Outport  InitialOutput=0
  !Q : Outport  Port=2  InitialOutput=1
  wires:
  Mux/1 -> Logic/1
  Logic/1 -> Demux/1
  Demux/2 -> !Q/1
  Demux/1 -> Q/1, Unit Delay/1
  Unit Delay/1 -> Mux/1
  S/1 -> Mux/2
  R/1 -> Mux/3

== system AC_Voltage_Control_3phase_IM/Subsystem1/Subsystem/P3/6 Flip-Flop/S-R Flip-Flop1 ==
  S : Inport
  R : Inport  Port=2
  Demux : Demux  Outputs=2
      settings: DisplayOption=none
  Logic : CombinatorialLogic  TruthTable=[0 1;0 1;1 0;0 1;1 0;0 1;1 0;1 0]
  Mux : Mux  Inputs=3
  Unit Delay : UnitDelay  InitialCondition=initial_condition  SampleTime=Ts
  Q : Outport  InitialOutput=0
  !Q : Outport  Port=2  InitialOutput=1
  wires:
  Mux/1 -> Logic/1
  Logic/1 -> Demux/1
  Demux/2 -> !Q/1
  Demux/1 -> Q/1, Unit Delay/1
  Unit Delay/1 -> Mux/1
  S/1 -> Mux/2
  R/1 -> Mux/3

== system AC_Voltage_Control_3phase_IM/Subsystem1/Subsystem/P4/6 Flip-Flop/S-R Flip-Flop1 ==
  S : Inport
  R : Inport  Port=2
  Demux : Demux  Outputs=2
      settings: DisplayOption=none
  Logic : CombinatorialLogic  TruthTable=[0 1;0 1;1 0;0 1;1 0;0 1;1 0;1 0]
  Mux : Mux  Inputs=3
  Unit Delay : UnitDelay  InitialCondition=initial_condition  SampleTime=Ts
  Q : Outport  InitialOutput=0
  !Q : Outport  Port=2  InitialOutput=1
  wires:
  R/1 -> Mux/3
  S/1 -> Mux/2
  Unit Delay/1 -> Mux/1
  Demux/1 -> Unit Delay/1, Q/1
  Demux/2 -> !Q/1
  Logic/1 -> Demux/1
  Mux/1 -> Logic/1

== system AC_Voltage_Control_3phase_IM/Subsystem1/Subsystem/P5/6 Flip-Flop/S-R Flip-Flop1 ==
  S : Inport
  R : Inport  Port=2
  Demux : Demux  Outputs=2
      settings: DisplayOption=none
  Logic : CombinatorialLogic  TruthTable=[0 1;0 1;1 0;0 1;1 0;0 1;1 0;1 0]
  Mux : Mux  Inputs=3
  Unit Delay : UnitDelay  InitialCondition=initial_condition  SampleTime=Ts
  Q : Outport  InitialOutput=0
  !Q : Outport  Port=2  InitialOutput=1
  wires:
  R/1 -> Mux/3
  S/1 -> Mux/2
  Unit Delay/1 -> Mux/1
  Demux/1 -> Unit Delay/1, Q/1
  Demux/2 -> !Q/1
  Logic/1 -> Demux/1
  Mux/1 -> Logic/1

== system AC_Voltage_Control_3phase_IM/Subsystem1/Subsystem/P6/6 Flip-Flop/S-R Flip-Flop1 ==
  S : Inport
  R : Inport  Port=2
  Demux : Demux  Outputs=2
      settings: DisplayOption=none
  Logic : CombinatorialLogic  TruthTable=[0 1;0 1;1 0;0 1;1 0;0 1;1 0;1 0]
  Mux : Mux  Inputs=3
  Unit Delay : UnitDelay  InitialCondition=initial_condition  SampleTime=Ts
  Q : Outport  InitialOutput=0
  !Q : Outport  Port=2  InitialOutput=1
  wires:
  Mux/1 -> Logic/1
  Logic/1 -> Demux/1
  Demux/2 -> !Q/1
  Demux/1 -> Q/1, Unit Delay/1
  Unit Delay/1 -> Mux/1
  S/1 -> Mux/2
  R/1 -> Mux/3
